simulink model "SolarPVACWithBattery_segmented1"  (R2024a)
settings: Solver=ode23t  StartTime=0.0  StopTime=25  MaxStep=1/(5*solarPlant.converterSwitchingFrequency)  RelTol=1e-3  AbsTol=1e-3
PreLoadFcn:
  | run('SolarPVACWithBatteryData');
undefined symbols (not defined in the file): bms, boost, dcVoltage, maxSoC, maxVdc, minIrrad, minSoC, minVdc, mppttime, olTime, sensor, sigbuilder_block, solarPlant
libraries: simulink x29, nesl_utility x21, fl_lib x19, ee_lib x15, eePwmGenerator x7, SignalEditorBlockLib x2, dspfdesign x1, batteryecm_lib x1, simulink_extras x1
(part 1 of 3)
Description:
  | Stand-Alone Solar PV AC Power System with Battery Backup
  | 
  | %
settings Model: Creator=The MathWorks, Inc.
settings SolverCC: AutoScaleAbsTol=off  ZeroCrossAlgorithm=Adaptive  AlgebraicLoopSolver=TrustRegion  MaxZcPerStep=1
settings DataIOCC: SaveOutput=off  DSMLogging=off  SaveTime=off  ReturnWorkspaceOutputs=off  SignalLoggingName=SolarPVACWithBattery_logDB
settings OptimizationCC: ReuseModelBlockBuffer=off
settings DebuggingCC: IgnoredZcDiagnostic=none  UnconnectedInputMsg=warning  UnconnectedOutputMsg=warning  UnconnectedLineMsg=warning  SymbolicDimsDataTypeCodeGenerationDiagnostic=none
settings ModelReferenceCC: EnableRefExpFcnMdlSchedulingChecks=on
settings SFSimCC: CustomCodeUndefinedFunction=UseInterfaceOnly
settings RTWCC: GPUComputeCapability=3.5  DLArmComputeVersion=19.05
settings SimscapeCC: SimscapeLogType=all  SimscapeLogSimulationStatistics=on  SimscapeLogName=simlog_SolarPVACWithBattery  SimscapeLogDataHistory=10000

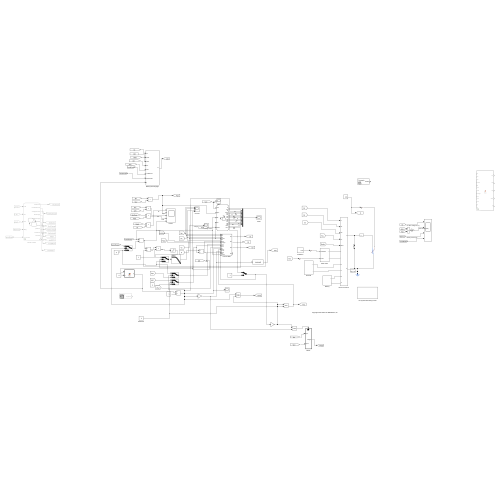
[thumbnail: Simulink's stored preview of the top-level diagram]
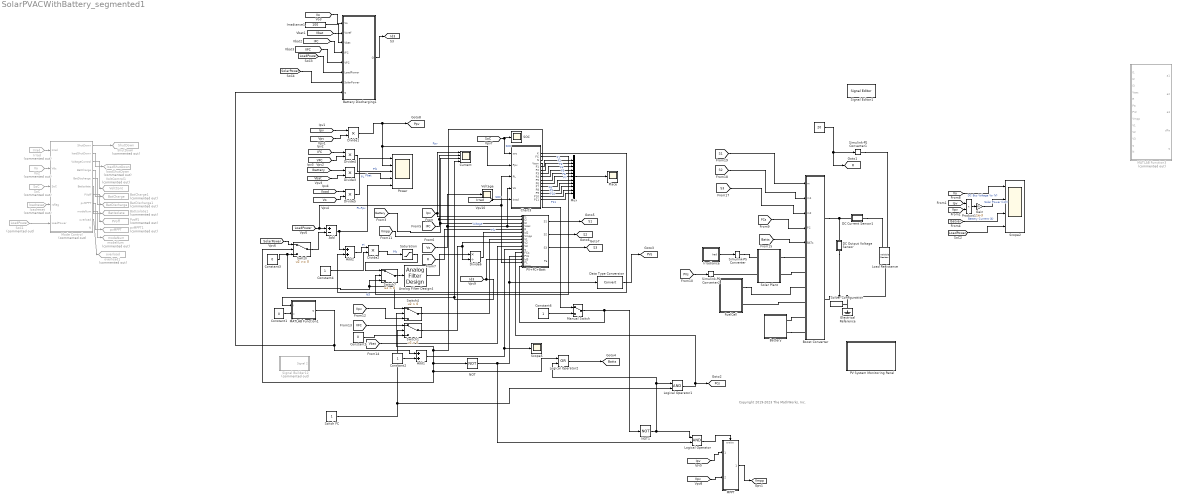
== system SolarPVACWithBattery_segmented1 ==
  note: Copyright 2019-2023 The MathWorks, Inc.
  " " : Constant  Value=20
  Add : Sum  Inputs=+-
  Add1 : Sum
  Add2 : Sum
  Analog Filter Design4 : dspfdesign/Analog Filter Design  method=Butterworth  filttype=Lowpass  N=2  Wlo=2  Whi=80  Rp=2  Rs=40
  BatCharge1 : Goto  Commented=on  GotoTag=BatCharge  TagVisibility=global
  BatDischarge1 : Goto  Commented=on  GotoTag=BatDischarge  TagVisibility=global
  BatIsolate1 : Goto  Commented=on  GotoTag=BatIsolate  TagVisibility=global
  Battery : Subsystem
  Battery Discharging1 : Subsystem
  Boost Converter : Subsystem  VariantControl=boostCircuit == 1
  Chart3 : Stateflow chart  TreatAsAtomicUnit=on
  Constant1 : Constant  Value=0
  Constant2 : Constant
  Constant3 : Constant  Value=0
  Constant4 : Constant
  Constant5 : Constant  Value=0
  Constant6 : Constant
  Current : Scope  NumInputPorts=4
  DC Current Sensor1 : Subsystem
      mask Display: disp('i')
  DC Output Voltage Sensor : Subsystem
      mask Display: disp('v')
  Data Type Conversion : DataTypeConversion  SaturateOnIntegerOverflow=off  RndMeth=Floor
  Divide{1..5} (5 alike) : Product  Inputs=**
  Divide6 : Product  Inputs=*/
  Electrical Reference : fl_lib/Electrical/Electrical Elements/Electrical Reference
  FuelCell : Subsystem
  Gain : Gain  Gain=1e-3
  Irrad : From  Commented=on  GotoTag=Irrad  TagVisibility=global
  Irradiance : Subsystem
  Irradiance1 : Constant  Value=100
  Load Resistance : fl_lib/Electrical/Electrical Elements/Variable Resistor  Rmin=0 Ohm  thermalEnable=false  thermal_mass=1 J/K  i_specify=off  i_priority=None  i=5 A  i_nominal_specify=off  i_nominal_value=1  i_nominal_unit=A  v_specify=off  v_priority=None  v=0 V  v_nominal_specify=off  v_nominal_value=1  v_nominal_unit=V  T_specify=off  T_priority=None  T=300 K  T_nominal_specify=off  T_nominal_value=1  T_nominal_unit=K
  Logical Operator : Logic  AllPortsSameDT=off  OutDataTypeStr=boolean
  Logical Operator1 : Logic  AllPortsSameDT=off  OutDataTypeStr=boolean
  Logical Operator2 : Logic  Operator=OR  AllPortsSameDT=off  OutDataTypeStr=boolean
  MATLAB Function1 : MATLAB Function  TreatAsAtomicUnit=on
  MATLAB Function3 : MATLAB Function  Commented=on  TreatAsAtomicUnit=on
  MPPT : Subsystem
  Manual Switch : ManualSwitch
  Mode Control : Stateflow chart  Commented=on  TreatAsAtomicUnit=on
  Mux : Mux  Inputs=11
  NOT : Logic  Operator=NOT  IconShape=distinctive  AllPortsSameDT=off  OutDataTypeStr=boolean
  NOT1 : Logic  Operator=NOT  IconShape=distinctive  AllPortsSameDT=off  OutDataTypeStr=boolean
  PV System Monitoring Panel : Subsystem
  PV+FC+Batt : Subsystem
  Place : Scope
  Power : Scope  NumInputPorts=5
  Product1 : Product
  Pvoff1 : Goto  Commented=on  GotoTag=PVoff  TagVisibility=global
  SOC : Scope
  Saturation : Saturate  UpperLimit=inf  LowerLimit=100
  Scope2 : Scope  NumInputPorts=4
  Scope5 : Scope
  ShutDown : Goto  Commented=on  GotoTag=ShutDown  TagVisibility=global
  Signal Builder12 : Subsystem  Tag=STV Subsys  Commented=on  LoadFcn=sigbuilder_block('load');  StartFcn=sigbuilder_block('start');  StopFcn=sigbuilder_block('stop');  ClipboardFcn=sigbuilder_block('clipboard');  mask(Sigbuilder block){tuvar=[0:10]}
      mask help: Simulink:masks:SigbuilderBlock_MD
      mask init:
      | if ~strcmp(get_param(bdroot(gcbh),'SimulationStatus'),'stopped') tuvar = sigbuilder_block('maskInit'); end
      settings: CopyFcn=sigbuilder_block('copy');  DeleteFcn=sigbuilder_block('delete');  ModelCloseFcn=sigbuilder_block('modelClose');  PreSaveFcn=sigbuilder_block('preSave');  PauseFcn=sigbuilder_block('pause');  ContinueFcn=sigbuilder_block('continue');  NameChangeFcn=sigbuilder_block('namechange');  OpenFcn=sigbuilder_block('open',[439.273 196.364 550.545 400 ]);  CloseFcn=sigbuilder_block('close');
      mask Display: plot(0, 0, 100, 100,[2, 2, 32, 32, 2], [68, 8, 8, 68, 68],[32, 2], [38, 38], [32, 19, 2],[53, 60, 44], [32, 17, 17, 2],[16, 16, 31, 31]);txt = getActiveGroup(gcbh);text(2, 100, txt,'verticalAlignment', 'top');
  Signal Editor1 : SignalEditorBlockLib/Signal Editor  FileName=signal.mat  ActiveScenario=Scenario  ActiveSignal=Pulse  IsBus=off  OutputBusObjectStr=Bus: BusObject  SampleTime=0  Interpolate=off  ZeroCross=off  OutputAfterFinalValue=Setting to zero  Unit=inherit  PreserveSignalName=on  ApplySigPropsToAllScenarios=on  ApplySigPropsToAllSignals=off
  Simulink-PS Converter : nesl_utility/Simulink-PS Converter  PhysicalDomain=network_engine_domain  SubClassName=ps_input  LeftPortType=input  RightPortType=output  PseudoPeriodic=off  Frequencies=[]  NoiseDistribution=none  NoiseParameters=[]  Unit=1  AffineConversion=off  FilteringAndDerivatives=provide  SimscapeFilterOrder=1  InputFilterTimeConstant=0.001  UdotUserProvided=0
  Simulink-PS Converter1 : nesl_utility/Simulink-PS Converter  PhysicalDomain=network_engine_domain  SubClassName=ps_input  LeftPortType=input  RightPortType=output  PseudoPeriodic=off  Frequencies=[]  NoiseDistribution=none  NoiseParameters=[]  Unit=1  AffineConversion=off  FilteringAndDerivatives=provide  SimscapeFilterOrder=1  InputFilterTimeConstant=0.001  UdotUserProvided=0
  Simulink-PS Converter2 : nesl_utility/Simulink-PS Converter  PhysicalDomain=network_engine_domain  SubClassName=ps_input  LeftPortType=input  RightPortType=output  PseudoPeriodic=off  Frequencies=[]  NoiseDistribution=none  NoiseParameters=[]  Unit=1  AffineConversion=off  FilteringAndDerivatives=provide  SimscapeFilterOrder=1  InputFilterTimeConstant=0.001  UdotUserProvided=0
  SoC : From  Commented=on  GotoTag=SoC  TagVisibility=global
  SoC1 : From  Commented=on  GotoTag=LoadPower  TagVisibility=global
  Solar Plant : Subsystem
  Solver Configuration : nesl_utility/Solver Configuration  PhysicalDomain=network_engine_domain  SubClassName=solver  LeftPortType=input  RightPortType=generic  Tones=[]  Harmonics=[]  SimulateNoise=off  Profile=off  UseLocalSampling=off  EnableSwitchedLinearOptims=on  FrequencyDomain=off  UseCCode=off  RelTol=0.001  AbsTol=1e-06  MinStep=1e-09  ToWorkspace=off  RevertToSquareIcSolve=off  NumHomotopyIterations=100  PhasorMode=off  PhasorModeNumHarmonics=1  ConsistencySolver=NEWTON_FTOL  IndexReductionMethod=DerivativeReplacement  DoDC=off  ResidualTolerance=1e-9  ConsistencyTolSource=GLOBAL  ConsistencyAbsTol=0.001  ConsistencyRelTol=0.001  ConsistencyTolFactor=0.001  UseLocalSolver=off  LocalSolverChoice=NE_BACKWARD_EULER_ADVANCER  ResolveIndetEquations=on  FunctionEvalNumThread=1  LocalSolverSampleTime=2e-6  DoFixedCost=off  MaxNonlinIter=10  MaxModeIter=2  ComputeImpulses=off  ImpulseIterations=2  LinearAlgebra=auto  LinearAlgebraNumThread=0  EquationFormulation=NE_TIME_EF  DelaysMemoryBudget=1024  AutomaticFiltering=on  FilteringTimeConstant=0.001  PartitionStorageMethod=AS_NEEDED  PartitionMemoryBudget=1024  PartitionMethod=FAST  MultibodyUseLocalSolver=off  MultibodyLocalSolverChoice=ODE1  MultibodyLocalSolverSampleTime=0.001
  Switch : Switch  SaturateOnIntegerOverflow=off  InputSameDT=off
  Switch1 : Switch  Criteria=u2 > Threshold  SaturateOnIntegerOverflow=off  InputSameDT=off
  Switch4 : Switch  Criteria=u2 > Threshold  SaturateOnIntegerOverflow=off  InputSameDT=off
  Switch7 : Switch  Criteria=u2 > Threshold  SaturateOnIntegerOverflow=off  InputSameDT=off
  Szitch FC : Constant
  Vo2 : From  Commented=on  GotoTag=Vo  TagVisibility=global
  VoltControl1 : Goto  Commented=on  GotoTag=VoltCont  TagVisibility=global
  Voltage : Scope
  loadShutDown : Goto  Commented=on  GotoTag=loadShutDown  TagVisibility=global
  loadreset : From  Commented=on  GotoTag=loadreset  TagVisibility=global
  modeNum : Goto  Commented=on  GotoTag=modeNum  TagVisibility=global
  overload1 : Goto  Commented=on  GotoTag=overload  TagVisibility=global
  pvMPPT1 : Goto  Commented=on  GotoTag=pvMPPT  TagVisibility=global
  tag scope: Batts=global, FCs=global, Id3=global, PVs=global, Ppv=global, R=global, S1=global, S2=global, S3=global, Vmpp=global
  wires:
  Mode Control/3(VoltageControl) -> VoltControl1/1
  [Vo] -> Scope2/1  "DC Bus Voltage Vo (V)"
  Product1/1 -> Gain/1
  Mode Control/4(BatCharge) -> BatCharge1/1
  Gain/1 -> Scope2/2  "Solar Power (kW)"
  Mode Control/7(PVoff) -> Pvoff1/1
  Mode Control/9(modeNum) -> modeNum/1
  Mode Control/1(ShutDown) -> ShutDown/1
  Mode Control/2(loadShutDown) -> loadShutDown/1
  Vo2/1 -> Mode Control/2(Vdc)
  [Ibatval] -> Scope2/3  "Battery Current (A)"
  loadreset/1 -> Mode Control/4(rsflag)
  SoC/1 -> Mode Control/3(SoC)
  Mode Control/10(overload) -> overload1/1
  [Vpv] -> Product1/2
  Irrad/1 -> Mode Control/1(Irrad)
  Mode Control/8(pvMPPT) -> pvMPPT1/1
  Mode Control/5(BatDischarge) -> BatDischarge1/1
  Mode Control/6(BatIsolate) -> BatIsolate1/1
  Irradiance/1(Irad) -> Simulink-PS Converter/1
  [Ipv] -> Product1/1
  " "/1 -> [R], Simulink-PS Converter1/1
  SoC1/1 -> Mode Control/5(LoadPower)
  [LoadPower] -> Scope2/4
  [R] -> PV+FC+Batt/5(R)
  [Vo] -> Voltage/1, Chart3/4(Vo), PV+FC+Batt/4(Vcac)  "Voltage"
  [Ipv] -> PV+FC+Batt/1(I1), Current/1
  [Vbat] -> PV+FC+Batt/10(V3)
  [IFC] -> Current/2, PV+FC+Batt/2(I2)
  Switch4/1 -> PV+FC+Batt/8(V1)
  [Vmpp] -> PV+FC+Batt/7(Vmpp)
  [IFC] -> Divide4/1
  [VFC] -> Divide4/2
  [Iload] -> Divide5/1
  [Ipv] -> Divide1/1
  [Vpv] -> Divide1/2
  [Vbat] -> Divide3/2
  Divide1/1 -> Chart3/2(Ppv), Power/2, [Ppv]  "Ppv"
  [Vo] -> Divide5/2
  [LoadPower] -> Add/1, Chart3/3(PL), PV+FC+Batt/15(PL)
  Switch/1 -> Add/2
  Analog Filter Design4/1 -> Divide6/1
  Add/1 -> Power/5, Add2/1  "PL-Ppv"
  Add1/1 -> PV+FC+Batt/11(q), Scope5/1
  Constant2/1 -> Add1/2
  [Ibattery] -> Current/3, PV+FC+Batt/3(I3)
  Constant1/1 -> MATLAB Function1/2(x)
  [SoC] -> Chart3/1(soc), SOC/1  "SOC"
  Divide5/1 -> Power/1  "PL"
  Divide4/1 -> Power/3  "Pfc"
  Divide3/1 -> Power/4  "Pbat"
  Add2/1 -> Divide2/1  "Pl"
  [S2] -> Boost Converter/2(m1)
  [S3] -> Boost Converter/3(m2)
  Constant3/1 -> Switch/3, Switch7/3, Switch4/1
  Chart3/3(N) -> Switch/2, Logical Operator2/1, NOT/1, Switch4/2
  [SolarPower] -> Switch/1
  Constant4/1 -> Divide2/2
  Divide2/1 -> Saturation/1  "Pfc"
  PV+FC+Batt/3(S3) -> [S3]
  PV+FC+Batt/2(S2) -> [S2]
  PV+FC+Batt/1(S1) -> [S1]
  Chart3/2(FC) -> Switch7/2
  Szitch FC/1 -> Logical Operator1/2, Switch1/2
  Saturation/1 -> Switch7/1
  Switch7/1 -> Analog Filter Design4/1
  [Vpv] -> Switch4/3
  [S1] -> Boost Converter/1(m)
  Switch1/1 -> PV+FC+Batt/9(V2), Divide6/2
  [VFC] -> Switch1/1
  Constant5/1 -> Switch1/3
  [Ipv] -> MPPT/1(Ipv1)
  [Vpv] -> MPPT/2(Vpv1)
  MPPT/1(Vmpp1) -> [Vmpp]
  NOT1/1 -> Logical Operator/1, Logical Operator1/1, Logical Operator2/2
  Chart3/4(Vcon) -> Manual Switch/1
  Logical Operator/1 -> MPPT/Enable
  [SolarPower] -> Battery Discharging1/7(SolarPower)
  Irradiance1/1 -> Battery Discharging1/2(Voref)
  [LoadPower] -> Battery Discharging1/6(LoadPower)
  Battery Discharging1/1(G) -> [Id3]
  [Vo] -> Battery Discharging1/1(Vo)
  [IFC] -> Battery Discharging1/4(IFC)
  [VFC] -> Battery Discharging1/5(VFC)
  [Vbat] -> Battery Discharging1/3(Vbat)
  MATLAB Function1/1(q) -> Battery Discharging1/8(q), Add1/1
  [Id3] -> MATLAB Function1/1(i), Current/4, PV+FC+Batt/14(Id3)  "Id3"
  [Ibattery] -> Divide3/1
  Divide6/1 -> PV+FC+Batt/6(Id2)  "Pfc"
  NOT/1 -> Data Type Conversion/1, PV+FC+Batt/13(PVs), Logical Operator/2
  Logical Operator1/1 -> PV+FC+Batt/12(FCs), [FCs]
  [PVs] -> Simulink-PS Converter2/1
  [FCs] -> Boost Converter/4(FC)
  [Batts] -> Boost Converter/5(BATs)
  Data Type Conversion/1 -> [PVs]
  Logical Operator2/1 -> [Batts]
  Chart3/1(K) -> Add2/2
  [Irrad] -> Chart3/5(Irrad)  "SOC"
  Chart3/14(P10) -> Mux/10  "P10"
  Chart3/5(P1) -> Mux/1  "P1"
  Chart3/6(P2) -> Mux/2  "P2"
  Chart3/7(P3) -> Mux/3  "P3"
  Chart3/8(P4) -> Mux/4  "P4"
  Chart3/9(P5) -> Mux/5  "P5"
  Chart3/10(P6) -> Mux/6  "P6"
  Chart3/11(P7) -> Mux/7  "P7"
  Chart3/12(P8) -> Mux/8  "P8"
  Chart3/13(P9) -> Mux/9  "P9"
  Chart3/15(P11) -> Mux/11  "P11"
  Mux/1 -> Place/1
  Manual Switch/1 -> PV+FC+Batt/16(Vcon), NOT1/1
  Constant6/1 -> Manual Switch/2
  connections:
  Solar Plant/RConn1 -- Boost Converter/LConn1
  DC Current Sensor1/RConn1 -- DC Output Voltage Sensor/RConn1 -- Boost Converter/RConn1
  Boost Converter/LConn2 -- Solar Plant/RConn2
  Simulink-PS Converter/RConn1 -- Solar Plant/LConn1
  Boost Converter/RConn2 -- Solver Configuration/RConn1 -- Electrical Reference/LConn1 -- Load Resistance/RConn1 -- DC Output Voltage Sensor/LConn1
  Simulink-PS Converter1/RConn1 -- Load Resistance/LConn1
  DC Current Sensor1/LConn1 -- Load Resistance/LConn2
  FuelCell/RConn1 -- Boost Converter/LConn3
  Boost Converter/LConn4 -- FuelCell/RConn2
  Battery/RConn1 -- Boost Converter/LConn5
  Battery/RConn2 -- Boost Converter/LConn6
  Solar Plant/LConn2 -- Simulink-PS Converter2/RConn1

== system SolarPVACWithBattery_segmented1/Battery ==
  Battery1 : batteryecm_lib/Battery  Vnom=50 V  prm_dir=1  R1_dis=2 Ohm  R1_ch=2 Ohm  R1=0.01 Ohm  prm_AH=2  AH=11.6 hr*A  V1=47 V  AH1=11.6*0.3 hr*A  prm_R2=simscape.enum.battery.prm_R2.enabled  R2=2000 Ohm  Tmeas=298.15 K  charge_measurement_port=simscape.enum.battery.enable.yes  prm_dyn=1  Rp1=0.005 Ohm  tau1=30 s  Rp2=0.005 Ohm  tau2=30 s  Rp3=0.005 Ohm  tau3=30 s  Rp4=0.005 Ohm  tau4=30 s  Rp5=0.005 Ohm  tau5=30 s  prm_fade=1  N_fade=100  AH_fade=45 hr*A  R1_fade=2.02 Ohm  R1_ch_fade=2.02 Ohm  V1_fade=10.35 V  prm_age=1  prm_age_OCV=1  OCV_age=0.9  SOC_age=60  Tmeas_age=298.15 K  delta_time_age_vec=[0] d  temperature_age_vec=[273] K  OCV_scaling_age=2.2134e6  OCV_offset_age=1.632e6  temp_exp_age=0.515833569 V  t_exp_age=0.75  Vnom_T2=12 V  R1_T2=2.2 Ohm  R1_T2_dis=2.2 Ohm  R1_T2_ch=2.2 Ohm  V1_T2=11.4 V  R2_T2=2200 Ohm  Rp1_T2=0.005 Ohm  tau1_T2=30 s  Rp2_T2=0.005 Ohm  tau2_T2=30 s  Rp3_T2=0.005 Ohm  tau3_T2=30 s  Rp4_T2=0.005 Ohm  tau4_T2=30 s  Rp5_T2=0.005 Ohm  tau5_T2=30 s  Tmeas2=273.15 K  thermal_port=simscape.enum.thermaleffects.omit  thermal_mass=30000 J/K  i_specify=off  i_priority=None  i=0 A  i_nominal_specify=off  i_nominal_value=1  i_nominal_unit=A  v_specify=off  v_priority=None  v=0 V  v_nominal_specify=off  v_nominal_value=1  v_nominal_unit=V  charge_specify=on  charge_priority=High  charge=8 hr*A  charge_nominal_specify=off  charge_nominal_value=1  charge_nominal_unit=A*hr  num_cycles_specify=off  num_cycles_priority=High  num_cycles=0  num_cycles_nominal_specify=off  num_cycles_nominal_value=1  num_cycles_nominal_unit=1  temperature_specify=off  temperature_priority=High  temperature=298.15 K  temperature_nominal_specify=off  temperature_nominal_value=1  temperature_nominal_unit=K
      settings: InternalSimscapePortConfiguration="{\"Bottom\":[],\"Left\":[{\"id\":\"p\",\"label\":\"+\",\"type\":\"foundation.electrical.electrical\"},{\"id\":\"q\",\"label\":\"q\",\"type\":\"output\"}],\"Right\":[{\"id\":\"n\",\"label\":\"-\",\"type\":\"foundation.electrical.electrical\"}],\"Top\":[]}"
  Charge to Ahr : Gain  Gain=1/3600
  DC Battery Current Sensor1 : Subsystem
      mask Display: disp('i');
  DC Battery Current Sensor2 : Subsystem
      mask Display: disp('i');
  DC Battery Voltage Sensor : Subsystem
      mask Display: disp('v');
  PS-Simulink Converter : nesl_utility/PS-Simulink Converter  PhysicalDomain=network_engine_domain  SubClassName=ps_output  LeftPortType=input  RightPortType=output  PseudoPeriodic=off  Frequencies=[]  VectorFormat=1-D array  Unit=inherit  AffineConversion=off
  Sensor Dynamics : simulink_extras/Additional Linear/Transfer Fcn (with initial outputs)  N=[1]  D=[1/sensor.samplingFreq 1]  Y0=minSoC  U0=0
  + : PMIOPort  Side=Right
  - : PMIOPort  Port=2  Side=Right
  tag scope: SoC=global
  wires:
  PS-Simulink Converter/1 -> Charge to Ahr/1
  Sensor Dynamics/1 -> [SoC]
  Charge to Ahr/1 -> Sensor Dynamics/1
  connections:
  DC Battery Voltage Sensor/LConn1 -- -/RConn1 -- Battery1/RConn1
  Battery1/LConn2 -- PS-Simulink Converter/LConn1
  DC Battery Current Sensor1/LConn1 -- +/RConn1
  DC Battery Voltage Sensor/RConn1 -- DC Battery Current Sensor1/RConn1 -- DC Battery Current Sensor2/LConn1
  DC Battery Current Sensor2/RConn1 -- Battery1/LConn1

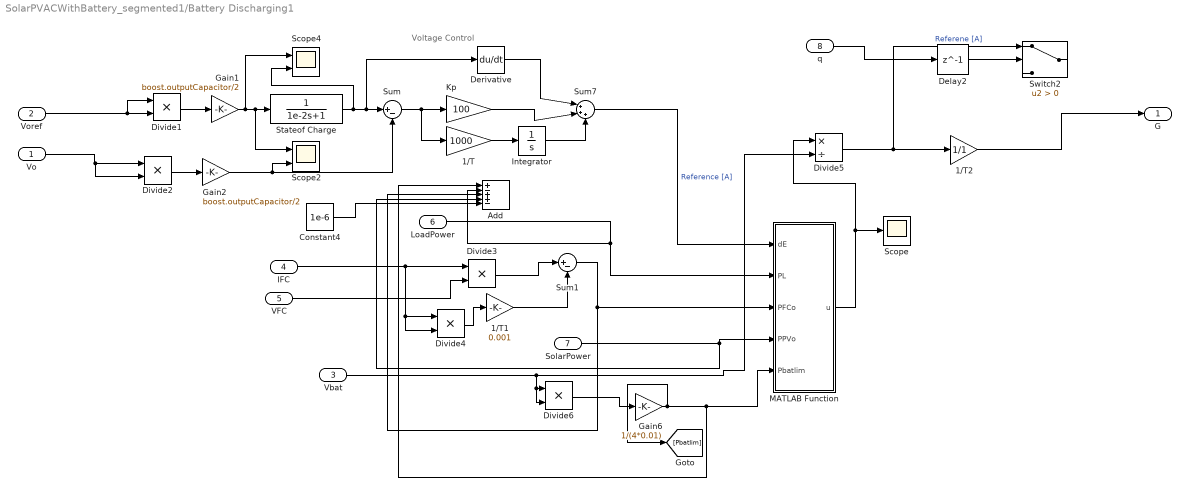
== system SolarPVACWithBattery_segmented1/Battery Discharging1 ==
  note: Voltage Control
  Vo : Inport
  Voref : Inport  Port=2
  Vbat : Inport  Port=3
  IFC : Inport  Port=4
  VFC : Inport  Port=5
  LoadPower : Inport  Port=6
  SolarPower : Inport  Port=7
  q : Inport  Port=8
  1/T : Gain  Gain=1000
  1/T1 : Gain  Gain=0.001
  1/T2 : Gain  Gain=1/1
  Add : Sum  Inputs=+-++-
  Constant4 : Constant  Value=1e-6
  Delay2 : Delay  DelayLength=1  InitialCondition=0
  Derivative : Derivative
  Divide{1..4,6} (5 alike) : Product  Inputs=**
  Divide5 : Product  Inputs=*/
  Gain1 : Gain  Gain=boost.outputCapacitor/2
  Gain2 : Gain  Gain=boost.outputCapacitor/2
  Gain6 : Gain  Gain=1/(4*0.01)
  Integrator : Integrator  UpperSaturationLimit=1500  LowerSaturationLimit=-1*1500
  Kp : Gain  Gain=100
  MATLAB Function : MATLAB Function  TreatAsAtomicUnit=on
  Scope : Scope
  Scope2 : Scope  NumInputPorts=2
  Scope4 : Scope  NumInputPorts=2
  Stateof Charge : TransferFcn  Denominator=[1e-2 1]
  Sum : Sum  Inputs=|+-
  Sum1 : Sum  Inputs=|+-
  Sum7 : Sum  Inputs=|+++
  Switch2 : Switch  Criteria=u2 > Threshold  SaturateOnIntegerOverflow=off  InputSameDT=off
  G : Outport
  wires:
  Divide3/1 -> Sum1/1
  Divide2/1 -> Gain2/1
  LoadPower/1 -> Add/2, MATLAB Function/2(PL)
  Integrator/1 -> Sum7/3
  Derivative/1 -> Sum7/1
  Divide6/1 -> Gain6/1
  Vo/1 -> Divide2/2, Divide2/1
  Sum1/1 -> Add/3, MATLAB Function/3(PFCo)
  Sum/1 -> 1/T/1, Kp/1
  VFC/1 -> Divide3/2
  Divide1/1 -> Gain1/1
  IFC/1 -> Divide4/2, Divide4/1, Divide3/1
  1/T/1 -> Integrator/1
  Gain6/1 -> [Pbatlim], Add/1, MATLAB Function/5(Pbatlim)
  MATLAB Function/1(u) -> Divide5/1, Scope/1
  SolarPower/1 -> Add/4, MATLAB Function/4(PPVo)
  Vbat/1 -> Divide5/2, Divide6/2, Divide6/1
  Gain2/1 -> Scope2/2, Sum/2
  Voref/1 -> Divide1/2, Divide1/1
  Divide4/1 -> 1/T1/1
  1/T1/1 -> Sum1/2
  Gain1/1 -> Scope4/1, Stateof Charge/1, Scope2/1
  Constant4/1 -> Add/5
  Kp/1 -> Sum7/2
  Stateof Charge/1 -> Scope4/2, Derivative/1, Sum/1
  Sum7/1 -> MATLAB Function/1(dE)  "Reference [A]"
  q/1 -> Delay2/1
  Divide5/1 -> 1/T2/1, Switch2/1  "Referene [A]"
  1/T2/1 -> G/1
  Delay2/1 -> Switch2/2

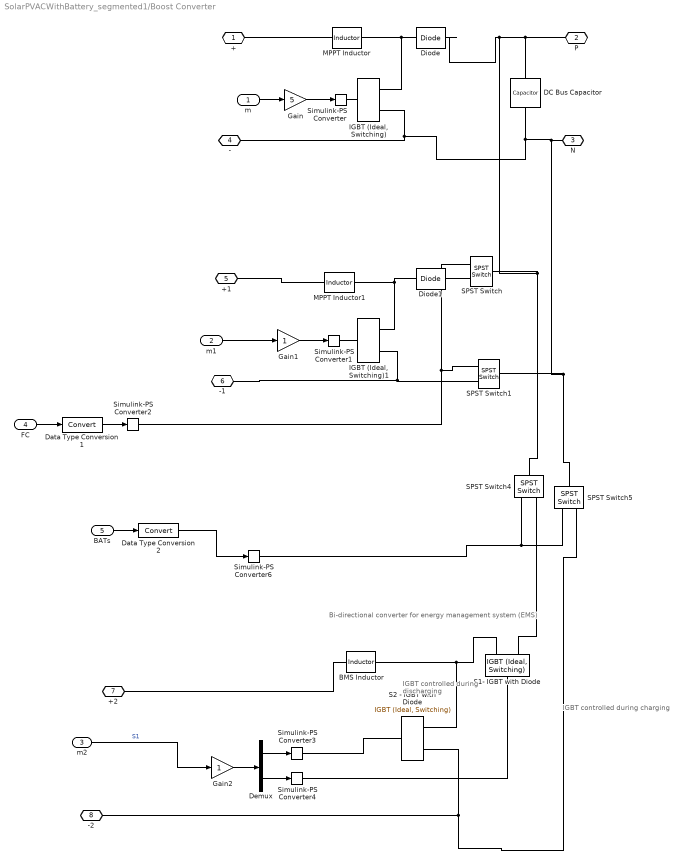
== system SolarPVACWithBattery_segmented1/Boost Converter ==
  note: Bi-directional converter for energy management system (EMS)
  note: IGBT controlled during charging
  note: IGBT controlled during discharging
  m : Inport
  m1 : Inport  Port=2
  m2 : Inport  Port=3
  FC : Inport  Port=4
  BATs : Inport  Port=5
  BMS Inductor : fl_lib/Electrical/Electrical Elements/Inductor  l=2e-3 H  r=0 Ohm  g=1e-9 1/Ohm  i_specify=off  i_priority=High  i=0 A  i_nominal_specify=off  i_nominal_value=1  i_nominal_unit=A  v_specify=off  v_priority=High  v=0 V  v_nominal_specify=off  v_nominal_value=1  v_nominal_unit=V  i_L_specify=on  i_L_priority=High  i_L=0 A  i_L_nominal_specify=off  i_L_nominal_value=1  i_L_nominal_unit=A
      settings: LogSimulationData=on
  DC Bus Capacitor : fl_lib/Electrical/Electrical Elements/Capacitor  c=0.015 F  r=0 Ohm  g=0 1/Ohm  i_specify=off  i_priority=None  i=0 A  i_nominal_specify=off  i_nominal_value=1  i_nominal_unit=A  v_specify=off  v_priority=None  v=0 V  v_nominal_specify=off  v_nominal_value=1  v_nominal_unit=V  vc_specify=on  vc_priority=High  vc=97 V  vc_nominal_specify=off  vc_nominal_value=1  vc_nominal_unit=V
  Data Type Conversion1 : DataTypeConversion  SaturateOnIntegerOverflow=off  RndMeth=Floor
  Data Type Conversion2 : DataTypeConversion  SaturateOnIntegerOverflow=off  RndMeth=Floor
  Demux : Demux  Outputs=2
  Diode : fl_lib/Electrical/Electrical Elements/Diode  Vf=0.8 V  Ron=1e-6 Ohm  Goff=1e-6 1/Ohm  i_specify=off  i_priority=None  i=0 A  i_nominal_specify=off  i_nominal_value=1  i_nominal_unit=A  v_specify=off  v_priority=None  v=0 V  v_nominal_specify=off  v_nominal_value=1  v_nominal_unit=V
  Diode1 : fl_lib/Electrical/Electrical Elements/Diode  Vf=0.8 V  Ron=1e-6 Ohm  Goff=1e-6 1/Ohm  i_specify=off  i_priority=None  i=0 A  i_nominal_specify=off  i_nominal_value=1  i_nominal_unit=A  v_specify=off  v_priority=None  v=0 V  v_nominal_specify=off  v_nominal_value=1  v_nominal_unit=V
  Gain : Gain  Gain=5
  Gain1 : Gain
  Gain2 : Gain
  "IGBT (Ideal, Switching)" : ee_lib/Semiconductors & Converters/IGBT (Ideal, Switching)  port_option=ee.enum.controlport.ps  Vf=0.1 V  Ron=1e-6 Ohm  Goff=1e-6 1/Ohm  Vth=0.5 V  diode_param=1  diode_Vf=0.8 V  diode_Ron=0.001 Ohm  diode_Goff=1e-5 1/Ohm  diode_C=50e-9 F  diode_iRM=-235 A  diode_iF=300 A  diode_idot=-50 A/us  diode_trr_param=1  diode_trr_factor=3  diode_trr=15 us  diode_Qrr=1500 s*uA  ice_specify=off  ice_priority=None  ice=0 A  ice_nominal_specify=off  ice_nominal_value=1  ice_nominal_unit=A  vce_specify=off  vce_priority=None  vce=0 V  vce_nominal_specify=off  vce_nominal_value=1  vce_nominal_unit=V  vge_specify=off  vge_priority=None  vge=0 V  vge_nominal_specify=off  vge_nominal_value=1  vge_nominal_unit=V  thermal_loss_option=ee.enum.converters.thermalLossOption.constantvalues  Von_data=[0, .1, .6, .8, 1, 1.3, 1.6, 2, 2.4; 0, .1, .7, 1, 1.2, 1.5, 1.9, 2.4, 2.8] V  Tj=[298.15, 398.15] K  Iout_data=[0, .1, 1, 5, 10, 20, 40, 70, 100] A  Eon_data=[0, .0024, .024, .12, .2, .48, 1.04, 2.16, 3.24; 0, .003, .03, .15, .25, .6, 1.3, 2.7, 4.05] * 1e-3 J  Eoff_data=[0, .0007, .0066, .033, .066, .17, .33, .83, 1.5; 0, .001, .01, .05, .1, .25, .5, 1.2, 2.2] * 1e-3 J  Eon_data_3D=[zeros(2, 9, 3)] J  Eoff_data_3D=[zeros(2, 9, 3)] J  Tj_loss=[298.15, 398.15] K  Iout_data_loss=[0, .1, 1, 5, 10, 20, 40, 70, 100] A  tabulateWithVce=false  Vce_loss=[0, 150, 300] V  Eon_scalar=22.86e-3 J  Eoff_scalar=17.14e-3 J  Voff=300 V  Iout_scalar=600 A  useCurrentFromPreviousCycle=false  useVoltageFromPreviousCycle=false  diodeModelType=ee.enum.converters.diodeModelType.pwl  diodeTableType=ee.enum.diode.tableType.IfMat  diode_ReverseIVType=ee.enum.diode.diodeReverseIV.constant  diode_IfMat=[.07, .12, .19, 1.75, 4.24, 7.32, 11.2; .16, .3, .72, 2.14, 4.02, 6.35, 9.12] A  diode_VfMat=[.9, 1.15, 1.25, 1.5, 1.75, 2.17, 2.6, 2.85; .58, .68, .75, 1.1, 1.38, 1.77, 2.27, 2.7] V  diode_TjVec=[25, 125] degC  diode_VfVec=[.5, .7, .9, 1.3, 1.7, 2.1, 2.5] V  diode_IfVec=[.1, .2, .5, 1, 2, 4, 7, 10] A  diode_IrMat=[1e-06, 2e-06, 5e-06, 1e-05, 2.5e-05, 5e-05, .0001; 2e-06, 5e-06, 1e-05, 4e-05, 8e-05, .0002, .0005] A  diode_VrMat=[10, 100, 200, 250, 300, 325, 350; 10, 70, 160, 220, 270, 300, 320] V  diode_VrVec=[10, 20, 40, 50, 70, 80, 100] V  diode_IrVec=[1e-06, 2e-06, 5e-06, 1e-05, 2e-05, 5e-05, .0001] A  diode_Vr=-600 V  diode_Ls=150 nH  diode_Erec=0.03 J  diode_rec_loss_model=ee.enum.diode.reverseRecoveryModel.fixed  diode_ErecVal=0 J  diode_scaleWithIandV=true  diode_ErecMat=zeros(2, 3) J  diode_TjrecVec=[298.15, 398.15] K  diode_IfrecVec=[.1, 1, 10] A  diode_IrecVal=10 A  diode_VrecVal=10 V  diode_tFilter=1 / 1000 / 100 s  thermal_network_parameterization=ee.enum.thermalNetworkTopology.external  Rth=[.08, .5] K/W  Rth_Cauer=[.08, .1, .5] K/W  Rth_Foster=[.08, .14, .22, .16] K/W  thermal_mass_parameterization=ee.enum.thermalNetwork.timeconstant  thermal_mass=[.01, .5] J/K  thermal_mass_Cauer=[.01, .1, .5] J/K  thermal_mass_Foster=[.001, .005, .05, .5] J/K  thermal_time_constant=[.001, .2] s  thermal_time_constant_Cauer=[.001, .1, .2] s  thermal_time_constant_Foster=[7e-05, .0007, .01, .08] s  thermal_mass_initial_temperatures=[25, 25] degC  thermal_mass_initial_temperatures_Cauer=[25, 25, 25] degC  junction_thermal_mass=0.01 J/K  Tvec_initial_Foster=[25, 25, 25, 25] degC  no_thermal_network=0  junction_temperature_specify=off  junction_temperature_priority=None  junction_temperature=25 degC  junction_temperature_nominal_specify=off  junction_temperature_nominal_value=1  junction_temperature_nominal_unit=degC  Qj_specify=off  Qj_priority=None  Qj=0 W  Qj_nominal_specify=off  Qj_nominal_value=1  Qj_nominal_unit=W  accumulatedSwitchingLosses_specify=off  accumulatedSwitchingLosses_priority=None  accumulatedSwitchingLosses=0 J
  "IGBT (Ideal, Switching)1" : ee_lib/Semiconductors & Converters/IGBT (Ideal, Switching)  port_option=ee.enum.controlport.ps  Vf=0.1 V  Ron=1e-6 Ohm  Goff=1e-6 1/Ohm  Vth=0.5 V  diode_param=1  diode_Vf=0.8 V  diode_Ron=0.001 Ohm  diode_Goff=1e-5 1/Ohm  diode_C=50e-9 F  diode_iRM=-235 A  diode_iF=300 A  diode_idot=-50 A/us  diode_trr_param=1  diode_trr_factor=3  diode_trr=15 us  diode_Qrr=1500 s*uA  ice_specify=off  ice_priority=None  ice=0 A  ice_nominal_specify=off  ice_nominal_value=1  ice_nominal_unit=A  vce_specify=off  vce_priority=None  vce=0 V  vce_nominal_specify=off  vce_nominal_value=1  vce_nominal_unit=V  vge_specify=off  vge_priority=None  vge=0 V  vge_nominal_specify=off  vge_nominal_value=1  vge_nominal_unit=V  thermal_loss_option=ee.enum.converters.thermalLossOption.constantvalues  Von_data=[0, .1, .6, .8, 1, 1.3, 1.6, 2, 2.4; 0, .1, .7, 1, 1.2, 1.5, 1.9, 2.4, 2.8] V  Tj=[298.15, 398.15] K  Iout_data=[0, .1, 1, 5, 10, 20, 40, 70, 100] A  Eon_data=[0, .0024, .024, .12, .2, .48, 1.04, 2.16, 3.24; 0, .003, .03, .15, .25, .6, 1.3, 2.7, 4.05] * 1e-3 J  Eoff_data=[0, .0007, .0066, .033, .066, .17, .33, .83, 1.5; 0, .001, .01, .05, .1, .25, .5, 1.2, 2.2] * 1e-3 J  Eon_data_3D=[zeros(2, 9, 3)] J  Eoff_data_3D=[zeros(2, 9, 3)] J  Tj_loss=[298.15, 398.15] K  Iout_data_loss=[0, .1, 1, 5, 10, 20, 40, 70, 100] A  tabulateWithVce=false  Vce_loss=[0, 150, 300] V  Eon_scalar=22.86e-3 J  Eoff_scalar=17.14e-3 J  Voff=300 V  Iout_scalar=600 A  useCurrentFromPreviousCycle=false  useVoltageFromPreviousCycle=false  diodeModelType=ee.enum.converters.diodeModelType.pwl  diodeTableType=ee.enum.diode.tableType.IfMat  diode_ReverseIVType=ee.enum.diode.diodeReverseIV.constant  diode_IfMat=[.07, .12, .19, 1.75, 4.24, 7.32, 11.2; .16, .3, .72, 2.14, 4.02, 6.35, 9.12] A  diode_VfMat=[.9, 1.15, 1.25, 1.5, 1.75, 2.17, 2.6, 2.85; .58, .68, .75, 1.1, 1.38, 1.77, 2.27, 2.7] V  diode_TjVec=[25, 125] degC  diode_VfVec=[.5, .7, .9, 1.3, 1.7, 2.1, 2.5] V  diode_IfVec=[.1, .2, .5, 1, 2, 4, 7, 10] A  diode_IrMat=[1e-06, 2e-06, 5e-06, 1e-05, 2.5e-05, 5e-05, .0001; 2e-06, 5e-06, 1e-05, 4e-05, 8e-05, .0002, .0005] A  diode_VrMat=[10, 100, 200, 250, 300, 325, 350; 10, 70, 160, 220, 270, 300, 320] V  diode_VrVec=[10, 20, 40, 50, 70, 80, 100] V  diode_IrVec=[1e-06, 2e-06, 5e-06, 1e-05, 2e-05, 5e-05, .0001] A  diode_Vr=-600 V  diode_Ls=150 nH  diode_Erec=0.03 J  diode_rec_loss_model=ee.enum.diode.reverseRecoveryModel.fixed  diode_ErecVal=0 J  diode_scaleWithIandV=true  diode_ErecMat=zeros(2, 3) J  diode_TjrecVec=[298.15, 398.15] K  diode_IfrecVec=[.1, 1, 10] A  diode_IrecVal=10 A  diode_VrecVal=10 V  diode_tFilter=1 / 1000 / 100 s  thermal_network_parameterization=ee.enum.thermalNetworkTopology.external  Rth=[.08, .5] K/W  Rth_Cauer=[.08, .1, .5] K/W  Rth_Foster=[.08, .14, .22, .16] K/W  thermal_mass_parameterization=ee.enum.thermalNetwork.timeconstant  thermal_mass=[.01, .5] J/K  thermal_mass_Cauer=[.01, .1, .5] J/K  thermal_mass_Foster=[.001, .005, .05, .5] J/K  thermal_time_constant=[.001, .2] s  thermal_time_constant_Cauer=[.001, .1, .2] s  thermal_time_constant_Foster=[7e-05, .0007, .01, .08] s  thermal_mass_initial_temperatures=[25, 25] degC  thermal_mass_initial_temperatures_Cauer=[25, 25, 25] degC  junction_thermal_mass=0.01 J/K  Tvec_initial_Foster=[25, 25, 25, 25] degC  no_thermal_network=0  junction_temperature_specify=off  junction_temperature_priority=None  junction_temperature=25 degC  junction_temperature_nominal_specify=off  junction_temperature_nominal_value=1  junction_temperature_nominal_unit=degC  Qj_specify=off  Qj_priority=None  Qj=0 W  Qj_nominal_specify=off  Qj_nominal_value=1  Qj_nominal_unit=W  accumulatedSwitchingLosses_specify=off  accumulatedSwitchingLosses_priority=None  accumulatedSwitchingLosses=0 J
  MPPT Inductor : ee_lib/Passive/Inductor  l=0.0797 H  enable_L_tol=0  L_tol=5  tol_distribution=1  nSigma=4  r=0 Ohm  g=1e-9 1/Ohm  enable_operating_limits=0  operating_limit_action=2  max_working_current=1 A  power_rating=1 W  enable_faults=ee.enum.enable.no  fault_action=simscape.enum.assert.action.none  lambdaPercent=50  k_faulted=0.9999  turnsShort=0  openCct=0  groundShort=0  groundShortG=0 1/Ohm  tau_fault=1e-3 s  fault_trigger=ee.enum.faults.faultTrigger.temporal  t_fault=1 s  max_permissible_voltage=100 V  n_fail_on_voltage=1  max_permissible_current=1 A  t_fail_on_current=1 s  i_L_specify=on  i_L_priority=High  i_L=0 A  i_L_nominal_specify=off  i_L_nominal_value=1  i_L_nominal_unit=A  faulted_specify=off  faulted_priority=None  faulted=0
  MPPT Inductor1 : ee_lib/Passive/Inductor  l=0.2677 H  enable_L_tol=0  L_tol=5  tol_distribution=1  nSigma=4  r=0 Ohm  g=1e-9 1/Ohm  enable_operating_limits=0  operating_limit_action=2  max_working_current=1 A  power_rating=1 W  enable_faults=ee.enum.enable.no  fault_action=simscape.enum.assert.action.none  lambdaPercent=50  k_faulted=0.9999  turnsShort=0  openCct=0  groundShort=0  groundShortG=0 1/Ohm  tau_fault=1e-3 s  fault_trigger=ee.enum.faults.faultTrigger.temporal  t_fault=1 s  max_permissible_voltage=100 V  n_fail_on_voltage=1  max_permissible_current=1 A  t_fail_on_current=1 s  i_L_specify=on  i_L_priority=High  i_L=0 A  i_L_nominal_specify=off  i_L_nominal_value=1  i_L_nominal_unit=A  faulted_specify=off  faulted_priority=None  faulted=0
  S1- IGBT with Diode : ee_lib/Semiconductors & Converters/IGBT (Ideal, Switching)  port_option=ee.enum.controlport.ps  Vf=0.1 V  Ron=1e-6 Ohm  Goff=1e-6 1/Ohm  Vth=0.5 V  diode_param=2  diode_Vf=0.8 V  diode_Ron=1e-12 Ohm  diode_Goff=1e-12 1/Ohm  diode_C=50e-9 F  diode_iRM=-235 A  diode_iF=300 A  diode_idot=-50 A/us  diode_trr_param=1  diode_trr_factor=3  diode_trr=15 us  diode_Qrr=1500 s*uA  ice_specify=off  ice_priority=None  ice=0 A  ice_nominal_specify=off  ice_nominal_value=1  ice_nominal_unit=A  vce_specify=off  vce_priority=None  vce=0 V  vce_nominal_specify=off  vce_nominal_value=1  vce_nominal_unit=V  vge_specify=off  vge_priority=None  vge=0 V  vge_nominal_specify=off  vge_nominal_value=1  vge_nominal_unit=V  thermal_loss_option=ee.enum.converters.thermalLossOption.constantvalues  Von_data=[0, .1, .6, .8, 1, 1.3, 1.6, 2, 2.4; 0, .1, .7, 1, 1.2, 1.5, 1.9, 2.4, 2.8] V  Tj=[298.15, 398.15] K  Iout_data=[0, .1, 1, 5, 10, 20, 40, 70, 100] A  Eon_data=[0, .0024, .024, .12, .2, .48, 1.04, 2.16, 3.24; 0, .003, .03, .15, .25, .6, 1.3, 2.7, 4.05] * 1e-3 J  Eoff_data=[0, .0007, .0066, .033, .066, .17, .33, .83, 1.5; 0, .001, .01, .05, .1, .25, .5, 1.2, 2.2] * 1e-3 J  Eon_data_3D=[zeros(2, 9, 3)] J  Eoff_data_3D=[zeros(2, 9, 3)] J  Tj_loss=[298.15, 398.15] K  Iout_data_loss=[0, .1, 1, 5, 10, 20, 40, 70, 100] A  tabulateWithVce=false  Vce_loss=[0, 150, 300] V  Eon_scalar=22.86e-3 J  Eoff_scalar=17.14e-3 J  Voff=300 V  Iout_scalar=600 A  useCurrentFromPreviousCycle=false  useVoltageFromPreviousCycle=false  diodeModelType=ee.enum.converters.diodeModelType.pwl  diodeTableType=ee.enum.diode.tableType.IfMat  diode_ReverseIVType=ee.enum.diode.diodeReverseIV.constant  diode_IfMat=[.07, .12, .19, 1.75, 4.24, 7.32, 11.2; .16, .3, .72, 2.14, 4.02, 6.35, 9.12] A  diode_VfMat=[.9, 1.15, 1.25, 1.5, 1.75, 2.17, 2.6, 2.85; .58, .68, .75, 1.1, 1.38, 1.77, 2.27, 2.7] V  diode_TjVec=[25, 125] degC  diode_VfVec=[.5, .7, .9, 1.3, 1.7, 2.1, 2.5] V  diode_IfVec=[.1, .2, .5, 1, 2, 4, 7, 10] A  diode_IrMat=[1e-06, 2e-06, 5e-06, 1e-05, 2.5e-05, 5e-05, .0001; 2e-06, 5e-06, 1e-05, 4e-05, 8e-05, .0002, .0005] A  diode_VrMat=[10, 100, 200, 250, 300, 325, 350; 10, 70, 160, 220, 270, 300, 320] V  diode_VrVec=[10, 20, 40, 50, 70, 80, 100] V  diode_IrVec=[1e-06, 2e-06, 5e-06, 1e-05, 2e-05, 5e-05, .0001] A  diode_Vr=-600 V  diode_Ls=150 nH  diode_Erec=0.03 J  diode_rec_loss_model=ee.enum.diode.reverseRecoveryModel.fixed  diode_ErecVal=0 J  diode_scaleWithIandV=true  diode_ErecMat=zeros(2, 3) J  diode_TjrecVec=[298.15, 398.15] K  diode_IfrecVec=[.1, 1, 10] A  diode_IrecVal=10 A  diode_VrecVal=10 V  diode_tFilter=1 / 1000 / 100 s  thermal_network_parameterization=ee.enum.thermalNetworkTopology.external  Rth=[.08, .5] K/W  Rth_Cauer=[.08, .1, .5] K/W  Rth_Foster=[.08, .14, .22, .16] K/W  thermal_mass_parameterization=ee.enum.thermalNetwork.timeconstant  thermal_mass=[.01, .5] J/K  thermal_mass_Cauer=[.01, .1, .5] J/K  thermal_mass_Foster=[.001, .005, .05, .5] J/K  thermal_time_constant=[.001, .2] s  thermal_time_constant_Cauer=[.001, .1, .2] s  thermal_time_constant_Foster=[7e-05, .0007, .01, .08] s  thermal_mass_initial_temperatures=[25, 25] degC  thermal_mass_initial_temperatures_Cauer=[25, 25, 25] degC  junction_thermal_mass=0.01 J/K  Tvec_initial_Foster=[25, 25, 25, 25] degC  no_thermal_network=0  junction_temperature_specify=off  junction_temperature_priority=None  junction_temperature=25 degC  junction_temperature_nominal_specify=off  junction_temperature_nominal_value=1  junction_temperature_nominal_unit=degC  Qj_specify=off  Qj_priority=None  Qj=0 W  Qj_nominal_specify=off  Qj_nominal_value=1  Qj_nominal_unit=W  accumulatedSwitchingLosses_specify=off  accumulatedSwitchingLosses_priority=None  accumulatedSwitchingLosses=0 J
  S2 - IGBT with Diode : ee_lib/Semiconductors & Converters/IGBT (Ideal, Switching)  port_option=ee.enum.controlport.ps  Vf=0.1 V  Ron=1e-6 Ohm  Goff=1e-6 1/Ohm  Vth=0.5 V  diode_param=2  diode_Vf=0.8 V  diode_Ron=1e-12 Ohm  diode_Goff=1e-12 1/Ohm  diode_C=50e-9 F  diode_iRM=-235 A  diode_iF=300 A  diode_idot=-50 A/us  diode_trr_param=1  diode_trr_factor=3  diode_trr=15 us  diode_Qrr=1500 s*uA  ice_specify=off  ice_priority=None  ice=0 A  ice_nominal_specify=off  ice_nominal_value=1  ice_nominal_unit=A  vce_specify=off  vce_priority=None  vce=0 V  vce_nominal_specify=off  vce_nominal_value=1  vce_nominal_unit=V  vge_specify=off  vge_priority=None  vge=0 V  vge_nominal_specify=off  vge_nominal_value=1  vge_nominal_unit=V  thermal_loss_option=ee.enum.converters.thermalLossOption.constantvalues  Von_data=[0, .1, .6, .8, 1, 1.3, 1.6, 2, 2.4; 0, .1, .7, 1, 1.2, 1.5, 1.9, 2.4, 2.8] V  Tj=[298.15, 398.15] K  Iout_data=[0, .1, 1, 5, 10, 20, 40, 70, 100] A  Eon_data=[0, .0024, .024, .12, .2, .48, 1.04, 2.16, 3.24; 0, .003, .03, .15, .25, .6, 1.3, 2.7, 4.05] * 1e-3 J  Eoff_data=[0, .0007, .0066, .033, .066, .17, .33, .83, 1.5; 0, .001, .01, .05, .1, .25, .5, 1.2, 2.2] * 1e-3 J  Eon_data_3D=[zeros(2, 9, 3)] J  Eoff_data_3D=[zeros(2, 9, 3)] J  Tj_loss=[298.15, 398.15] K  Iout_data_loss=[0, .1, 1, 5, 10, 20, 40, 70, 100] A  tabulateWithVce=false  Vce_loss=[0, 150, 300] V  Eon_scalar=22.86e-3 J  Eoff_scalar=17.14e-3 J  Voff=300 V  Iout_scalar=600 A  useCurrentFromPreviousCycle=false  useVoltageFromPreviousCycle=false  diodeModelType=ee.enum.converters.diodeModelType.pwl  diodeTableType=ee.enum.diode.tableType.IfMat  diode_ReverseIVType=ee.enum.diode.diodeReverseIV.constant  diode_IfMat=[.07, .12, .19, 1.75, 4.24, 7.32, 11.2; .16, .3, .72, 2.14, 4.02, 6.35, 9.12] A  diode_VfMat=[.9, 1.15, 1.25, 1.5, 1.75, 2.17, 2.6, 2.85; .58, .68, .75, 1.1, 1.38, 1.77, 2.27, 2.7] V  diode_TjVec=[25, 125] degC  diode_VfVec=[.5, .7, .9, 1.3, 1.7, 2.1, 2.5] V  diode_IfVec=[.1, .2, .5, 1, 2, 4, 7, 10] A  diode_IrMat=[1e-06, 2e-06, 5e-06, 1e-05, 2.5e-05, 5e-05, .0001; 2e-06, 5e-06, 1e-05, 4e-05, 8e-05, .0002, .0005] A  diode_VrMat=[10, 100, 200, 250, 300, 325, 350; 10, 70, 160, 220, 270, 300, 320] V  diode_VrVec=[10, 20, 40, 50, 70, 80, 100] V  diode_IrVec=[1e-06, 2e-06, 5e-06, 1e-05, 2e-05, 5e-05, .0001] A  diode_Vr=-600 V  diode_Ls=150 nH  diode_Erec=0.03 J  diode_rec_loss_model=ee.enum.diode.reverseRecoveryModel.fixed  diode_ErecVal=0 J  diode_scaleWithIandV=true  diode_ErecMat=zeros(2, 3) J  diode_TjrecVec=[298.15, 398.15] K  diode_IfrecVec=[.1, 1, 10] A  diode_IrecVal=10 A  diode_VrecVal=10 V  diode_tFilter=1 / 1000 / 100 s  thermal_network_parameterization=ee.enum.thermalNetworkTopology.external  Rth=[.08, .5] K/W  Rth_Cauer=[.08, .1, .5] K/W  Rth_Foster=[.08, .14, .22, .16] K/W  thermal_mass_parameterization=ee.enum.thermalNetwork.timeconstant  thermal_mass=[.01, .5] J/K  thermal_mass_Cauer=[.01, .1, .5] J/K  thermal_mass_Foster=[.001, .005, .05, .5] J/K  thermal_time_constant=[.001, .2] s  thermal_time_constant_Cauer=[.001, .1, .2] s  thermal_time_constant_Foster=[7e-05, .0007, .01, .08] s  thermal_mass_initial_temperatures=[25, 25] degC  thermal_mass_initial_temperatures_Cauer=[25, 25, 25] degC  junction_thermal_mass=0.01 J/K  Tvec_initial_Foster=[25, 25, 25, 25] degC  no_thermal_network=0  junction_temperature_specify=off  junction_temperature_priority=None  junction_temperature=25 degC  junction_temperature_nominal_specify=off  junction_temperature_nominal_value=1  junction_temperature_nominal_unit=degC  Qj_specify=off  Qj_priority=None  Qj=0 W  Qj_nominal_specify=off  Qj_nominal_value=1  Qj_nominal_unit=W  accumulatedSwitchingLosses_specify=off  accumulatedSwitchingLosses_priority=None  accumulatedSwitchingLosses=0 J
  SPST Switch{,1,4..5} (4 alike) : ee_lib/Switches & Breakers/SPST Switch  R_closed=0.01 Ohm  G_open=1e-6 S  Threshold=0.5 V  Width=0 V  model_dynamics=0  t_on=1e-3 s  t_off=1e-3 s  initial_vT=0 V
      settings: InternalSimscapePortConfiguration="{\"Bottom\":[],\"Left\":[{\"id\":\"vT\",\"label\":\"vT\",\"type\":\"input\"},{\"id\":\"p\",\"label\":\"\",\"type\":\"foundation.electrical.electrical\"}],\"Right\":[{\"id\":\"n\",\"label\":\"\",\"type\":\"foundation.electrical.electrical\"}],\"Top\":[]}"
  Simulink-PS Converter{,1..4,6} (6 alike) : nesl_utility/Simulink-PS Converter  PhysicalDomain=network_engine_domain  SubClassName=ps_input  LeftPortType=input  RightPortType=output  PseudoPeriodic=off  Frequencies=[]  NoiseDistribution=none  NoiseParameters=[]  Unit=1  AffineConversion=off  FilteringAndDerivatives=provide  SimscapeFilterOrder=1  InputFilterTimeConstant=0.001  UdotUserProvided=0
  + : PMIOPort  Side=Left
  P : PMIOPort  Port=2  Side=Right
  N : PMIOPort  Port=3  Side=Right
  - : PMIOPort  Port=4  Side=Left
  +1 : PMIOPort  Port=5  Side=Left
  -1 : PMIOPort  Port=6  Side=Left
  +2 : PMIOPort  Port=7  Side=Left
  -2 : PMIOPort  Port=8  Side=Left
  wires:
  m/1 -> Gain/1
  Gain/1 -> Simulink-PS Converter/1
  Gain1/1 -> Simulink-PS Converter1/1
  m1/1 -> Gain1/1
  Data Type Conversion1/1 -> Simulink-PS Converter2/1
  FC/1 -> Data Type Conversion1/1
  Gain2/1 -> Demux/1
  Demux/2 -> Simulink-PS Converter4/1
  m2/1 -> Gain2/1  "S1"
  Demux/1 -> Simulink-PS Converter3/1
  Data Type Conversion2/1 -> Simulink-PS Converter6/1
  BATs/1 -> Data Type Conversion2/1
  connections:
  +/RConn1 -- MPPT Inductor/LConn1
  "IGBT (Ideal, Switching)"/LConn1 -- Simulink-PS Converter/RConn1
  MPPT Inductor/RConn1 -- "IGBT (Ideal, Switching)"/RConn1 -- Diode/LConn1
  "IGBT (Ideal, Switching)1"/RConn1 -- Diode1/LConn1 -- MPPT Inductor1/RConn1
  "IGBT (Ideal, Switching)1"/LConn1 -- Simulink-PS Converter1/RConn1
  MPPT Inductor1/LConn1 -- +1/RConn1
  Simulink-PS Converter2/RConn1 -- SPST Switch/LConn1 -- SPST Switch1/LConn1
  SPST Switch/RConn1 -- SPST Switch4/RConn1 -- Diode/RConn1 -- DC Bus Capacitor/LConn1 -- P/RConn1
  BMS Inductor/RConn1 -- S1- IGBT with Diode/RConn2 -- S2 - IGBT with Diode/RConn1
  Simulink-PS Converter4/RConn1 -- S1- IGBT with Diode/LConn1
  Simulink-PS Converter3/RConn1 -- S2 - IGBT with Diode/LConn1
  BMS Inductor/LConn1 -- +2/RConn1
  SPST Switch/LConn2 -- Diode1/RConn1
  "IGBT (Ideal, Switching)1"/RConn2 -- SPST Switch1/LConn2 -- -1/RConn1
  -2/RConn1 -- S2 - IGBT with Diode/RConn2 -- SPST Switch5/LConn2
  Simulink-PS Converter6/RConn1 -- SPST Switch4/LConn1 -- SPST Switch5/LConn1
  SPST Switch4/LConn2 -- S1- IGBT with Diode/RConn1
  DC Bus Capacitor/RConn1 -- -/RConn1 -- "IGBT (Ideal, Switching)"/RConn2 -- SPST Switch5/RConn1 -- SPST Switch1/RConn1 -- N/RConn1

== system SolarPVACWithBattery_segmented1/DC Current Sensor1 ==
  Current Sensor : fl_lib/Electrical/Electrical Sensors/Current Sensor
      settings: LogSimulationData=on
  PS-Simulink Converter : nesl_utility/PS-Simulink Converter  PhysicalDomain=network_engine_domain  SubClassName=ps_output  LeftPortType=input  RightPortType=output  PseudoPeriodic=off  Frequencies=[]  VectorFormat=1-D array  Unit=1  AffineConversion=off
  Sensor dynamics : TransferFcn  Numerator=1  Denominator=[1/sensor.samplingFreq 1]
  - : PMIOPort  Side=Left
  + : PMIOPort  Port=2  Side=Right
  tag scope: Iload=global
  wires:
  PS-Simulink Converter/1 -> Sensor dynamics/1
  Sensor dynamics/1 -> [Iload]
  connections:
  Current Sensor/RConn2 -- -/RConn1
  +/RConn1 -- Current Sensor/LConn1
  Current Sensor/RConn1 -- PS-Simulink Converter/LConn1

== system SolarPVACWithBattery_segmented1/DC Output Voltage Sensor ==
  PS-Simulink Converter : nesl_utility/PS-Simulink Converter  PhysicalDomain=network_engine_domain  SubClassName=ps_output  LeftPortType=input  RightPortType=output  PseudoPeriodic=off  Frequencies=[]  VectorFormat=1-D array  Unit=1  AffineConversion=off
  Sensor dynamics : TransferFcn  Numerator=1  Denominator=[1/sensor.samplingFreq 1]
  Voltage Sensor : fl_lib/Electrical/Electrical Sensors/Voltage Sensor
  - : PMIOPort  Side=Left
  + : PMIOPort  Port=2  Side=Right
  tag scope: Vo=global
  wires:
  PS-Simulink Converter/1 -> Sensor dynamics/1
  Sensor dynamics/1 -> [Vo]
  connections:
  Voltage Sensor/RConn2 -- -/RConn1
  Voltage Sensor/RConn1 -- PS-Simulink Converter/LConn1
  Voltage Sensor/LConn1 -- +/RConn1

== system SolarPVACWithBattery_segmented1/FuelCell ==
  " 2" : Constant  Commented=on
  Current Sensor : fl_lib/Electrical/Electrical Sensors/Current Sensor
      settings: LogSimulationData=on
  DC Voltage Source : fl_lib/Electrical/Electrical Sources/DC Voltage Source  v0=50 V
  Data Type Conversion1 : DataTypeConversion  Commented=on  SaturateOnIntegerOverflow=off  RndMeth=Floor
  Display : Display
  Display1 : Display
  Display2 : Display
  Fuel Cell : ee_lib/Sources/Fuel Cell  model_fidelity=ee.enum.fuelcell.fidelity.simplified  Eoc=50 V  A=0.01 V  ri=0.001 Ohm  i0=60 A  i_lim=200 A  N_cell=40  number_unit=1  pH2_nom=1.5e5 Pa  pO2_nom=1.0e5 Pa  xH2=99  xO2=21  xW=1  dyn=ee.enum.include.no  Rd=0.005 Ohm  tau=10 s  Tnom=293.15 K  thermal_mass=30000 J/K  iFC_specify=off  iFC_priority=None  iFC=0 A  iFC_nominal_specify=off  iFC_nominal_value=1  iFC_nominal_unit=A  vFC_specify=on  vFC_priority=High  vFC=50 V  vFC_nominal_specify=off  vFC_nominal_value=40  vFC_nominal_unit=V  temperature_specify=off  temperature_priority=High  temperature=293 K  temperature_nominal_specify=off  temperature_nominal_value=1  temperature_nominal_unit=K
      settings: InternalSimscapePortConfiguration="{\"Bottom\":[],\"Left\":[],\"Right\":[{\"id\":\"p\",\"label\":\"+\",\"type\":\"foundation.electrical.electrical\"},{\"id\":\"n\",\"label\":\"-\",\"type\":\"foundation.electrical.electrical\"}],\"Top\":[]}"
  PS-Simulink Converter : nesl_utility/PS-Simulink Converter  PhysicalDomain=network_engine_domain  SubClassName=ps_output  LeftPortType=input  RightPortType=output  PseudoPeriodic=off  Frequencies=[]  VectorFormat=1-D array  Unit=1  AffineConversion=off
  PS-Simulink Converter1 : nesl_utility/PS-Simulink Converter  PhysicalDomain=network_engine_domain  SubClassName=ps_output  LeftPortType=input  RightPortType=output  PseudoPeriodic=off  Frequencies=[]  VectorFormat=1-D array  Unit=1  AffineConversion=off
  Product : Product
  SPST Switch : ee_lib/Switches & Breakers/SPST Switch  Commented=on  R_closed=0.01 Ohm  G_open=1e-6 S  Threshold=0.5 V  Width=0 V  model_dynamics=0  t_on=1e-3 s  t_off=1e-3 s  initial_vT=0 V
      settings: InternalSimscapePortConfiguration="{\"Bottom\":[],\"Left\":[{\"id\":\"vT\",\"label\":\"vT\",\"type\":\"input\"},{\"id\":\"p\",\"label\":\"\",\"type\":\"foundation.electrical.electrical\"}],\"Right\":[{\"id\":\"n\",\"label\":\"\",\"type\":\"foundation.electrical.electrical\"}],\"Top\":[]}"
  SPST Switch1 : ee_lib/Switches & Breakers/SPST Switch  Commented=on  R_closed=0.01 Ohm  G_open=1e-6 S  Threshold=0.5 V  Width=0 V  model_dynamics=0  t_on=1e-3 s  t_off=1e-3 s  initial_vT=0 V
      settings: InternalSimscapePortConfiguration="{\"Bottom\":[],\"Left\":[{\"id\":\"vT\",\"label\":\"vT\",\"type\":\"input\"},{\"id\":\"p\",\"label\":\"\",\"type\":\"foundation.electrical.electrical\"}],\"Right\":[{\"id\":\"n\",\"label\":\"\",\"type\":\"foundation.electrical.electrical\"}],\"Top\":[]}"
  Sensor dynamics : TransferFcn  Numerator=1  Denominator=[1/sensor.samplingFreq 1]
  Sensor dynamics1 : TransferFcn  Numerator=1  Denominator=[1/sensor.samplingFreq 1]
  Simulink-PS Converter2 : nesl_utility/Simulink-PS Converter  Commented=on  PhysicalDomain=network_engine_domain  SubClassName=ps_input  LeftPortType=input  RightPortType=output  PseudoPeriodic=off  Frequencies=[]  NoiseDistribution=none  NoiseParameters=[]  Unit=1  AffineConversion=off  FilteringAndDerivatives=provide  SimscapeFilterOrder=1  InputFilterTimeConstant=0.001  UdotUserProvided=0
  Voltage Sensor : fl_lib/Electrical/Electrical Sensors/Voltage Sensor
      settings: LogSimulationData=on
  + : PMIOPort  Side=Right
  - : PMIOPort  Port=2  Side=Right
  tag scope: FCPower=global, IFC=global, VFC=global
  wires:
  Sensor dynamics/1 -> Product/1, Display/1
  PS-Simulink Converter1/1 -> Sensor dynamics1/1
  Sensor dynamics1/1 -> [VFC], Product/2, Display1/1
  PS-Simulink Converter/1 -> [IFC], Sensor dynamics/1
  Product/1 -> [FCPower], Display2/1  "FC power"
  Data Type Conversion1/1 -> Simulink-PS Converter2/1
  " 2"/1 -> Data Type Conversion1/1
  connections:
  Voltage Sensor/RConn2 -- Fuel Cell/RConn2 -- -/RConn1
  Voltage Sensor/LConn1 -- +/RConn1 -- Current Sensor/RConn2
  Current Sensor/RConn1 -- PS-Simulink Converter/LConn1
  Voltage Sensor/RConn1 -- PS-Simulink Converter1/LConn1
  Current Sensor/LConn1 -- Fuel Cell/RConn1

== system SolarPVACWithBattery_segmented1/Irradiance ==
  " " : Constant
  Sensor dynamics : TransferFcn  Numerator=1  Denominator=[1/sensor.samplingFreq 1]
  Signal Editor : SignalEditorBlockLib/Signal Editor  FileName=signal.mat  ActiveScenario=Scenario1  ActiveSignal=Pulse  IsBus=off  OutputBusObjectStr=Bus: BusObject  SampleTime=0  Interpolate=off  ZeroCross=off  OutputAfterFinalValue=Setting to zero  Unit=inherit  PreserveSignalName=on  ApplySigPropsToAllScenarios=on  ApplySigPropsToAllSignals=off
  Solar Irradiance W/m2 : Gain  Gain=1000
  Irad : Outport
  tag scope: Irrad=global
  wires:
  Solar Irradiance W/m2/1 -> Irad/1, Sensor dynamics/1
  Sensor dynamics/1 -> [Irrad]
  " "/1 -> Solar Irradiance W/m2/1

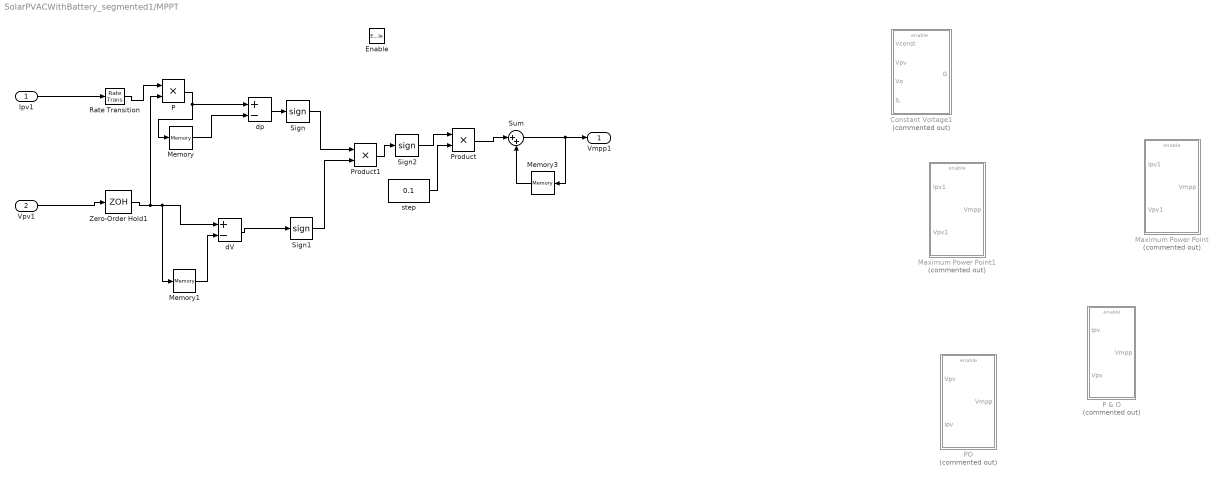
== system SolarPVACWithBattery_segmented1/MPPT ==
  Ipv1 : Inport
  Vpv1 : Inport  Port=2
  Enable : EnablePort  StatesWhenEnabling=reset
  Constant Voltage1 : Subsystem  Commented=on
  Maximum Power Point : Subsystem  Commented=on
  Maximum Power Point1 : Subsystem  Commented=on
  Memory : Memory  InheritSampleTime=on
  Memory1 : Memory  InheritSampleTime=on
  Memory3 : Memory  InitialCondition=50  InheritSampleTime=on
  P : Product  RndMeth=Zero
  P & O : Subsystem  Commented=on
  PO : Subsystem  Commented=on
  Product : Product  RndMeth=Zero
  Product1 : Product  RndMeth=Zero
  Rate Transition : RateTransition  OutPortSampleTime=mppttime
  Sign : Signum
  Sign1 : Signum
  Sign2 : Signum
  Sum : Sum  Inputs=|++
  Zero-Order Hold1 : ZeroOrderHold  SampleTime=mppttime
  dV : Sum  Inputs=+-
  dp : Sum  Inputs=+-
  step : Constant  Value=0.1
  Vmpp1 : Outport
  wires:
  Product1/1 -> Sign2/1
  Rate Transition/1 -> P/1
  Memory3/1 -> Sum/2
  Ipv1/1 -> Rate Transition/1
  Memory/1 -> dp/2
  Vpv1/1 -> Zero-Order Hold1/1
  Product/1 -> Sum/1
  P/1 -> Memory/1, dp/1
  dV/1 -> Sign1/1
  step/1 -> Product/2
  Zero-Order Hold1/1 -> P/2, dV/1, Memory1/1
  dp/1 -> Sign/1
  Sum/1 -> Memory3/1, Vmpp1/1
  Memory1/1 -> dV/2
  Sign2/1 -> Product/1
  Sign/1 -> Product1/1
  Sign1/1 -> Product1/2
